simulink model "Gen_nl"  (R2018b)
settings: Solver=FixedStepAuto  StartTime=0.0  StopTime=100  FixedStep=0.1  RelTol=1e-3
undefined symbols (not defined in the file): g, Jx, Jy, Jz, m, phi_DoS_duration, phi_FDI_value, phi_Replay_delay, psi_DoS_duration, psi_FDI_value, psi_Replay_delay, T_DoS_duration, T_FDI_value, T_Replay_delay, tau_phi_DoS_duration, tau_phi_FDI_value, tau_phi_Replay_delay, tau_psi_DoS_duration, tau_psi_FDI_value, tau_psi_Replay_delay, tau_theta_DoS_duration, tau_theta_FDI_value, tau_theta_Replay_delay, theta_DoS_duration, theta_FDI_value, theta_Replay_delay, x_DoS_duration, x_FDI_value, x_Replay_delay, y_DoS_duration, y_FDI_value, y_Replay_delay, z_DoS_duration, z_FDI_value, z_Replay_delay
libraries: simulink x6
settings Model: Creator=afsha  LastModifiedBy=afsha
settings DataIOCC: ReturnWorkspaceOutputs=on  ReturnWorkspaceOutputsName=logsout

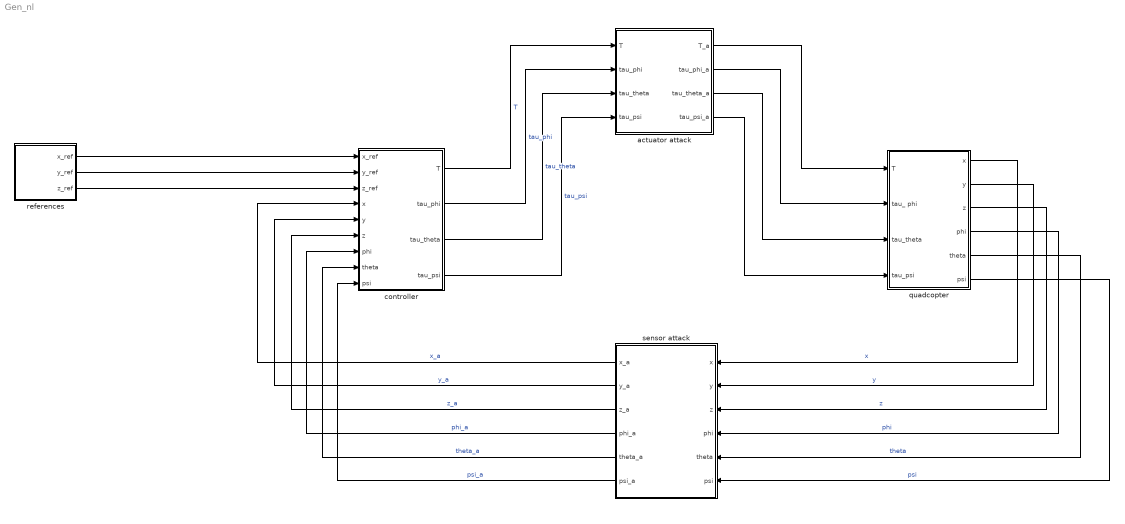
== system Gen_nl ==
  actuator attack : Subsystem
  controller : Subsystem
  quadcopter : Subsystem
  references : Subsystem
  sensor attack : Subsystem
  wires:
  quadcopter/1(x) -> sensor attack/1(x)  "x"
  quadcopter/2(y) -> sensor attack/2(y)  "y"
  quadcopter/3(z) -> sensor attack/3(z)  "z"
  quadcopter/4(phi) -> sensor attack/4(phi)  "phi"
  quadcopter/5(theta) -> sensor attack/5(theta)  "theta"
  quadcopter/6(psi) -> sensor attack/6(psi)  "psi"
  references/1(x_ref) -> controller/1(x_ref)
  references/2(y_ref) -> controller/2(y_ref)
  references/3(z_ref) -> controller/3(z_ref)
  controller/1(T) -> actuator attack/1(T)  "T"
  controller/2(tau_phi) -> actuator attack/2(tau_phi)  "tau_phi"
  controller/3(tau_theta) -> actuator attack/3(tau_theta)  "tau_theta"
  controller/4(tau_psi) -> actuator attack/4(tau_psi)  "tau_psi"
  actuator attack/1(T_a) -> quadcopter/1(T)
  actuator attack/2(tau_phi_a) -> quadcopter/2(tau_ phi)
  actuator attack/3(tau_theta_a) -> quadcopter/3(tau_theta)
  actuator attack/4(tau_psi_a) -> quadcopter/4(tau_psi)
  sensor attack/1(x_a) -> controller/4(x)  "x_a"
  sensor attack/2(y_a) -> controller/5(y)  "y_a"
  sensor attack/3(z_a) -> controller/6(z)  "z_a"
  sensor attack/4(phi_a) -> controller/7(phi)  "phi_a"
  sensor attack/5(theta_a) -> controller/8(theta)  "theta_a"
  sensor attack/6(psi_a) -> controller/9(psi)  "psi_a"

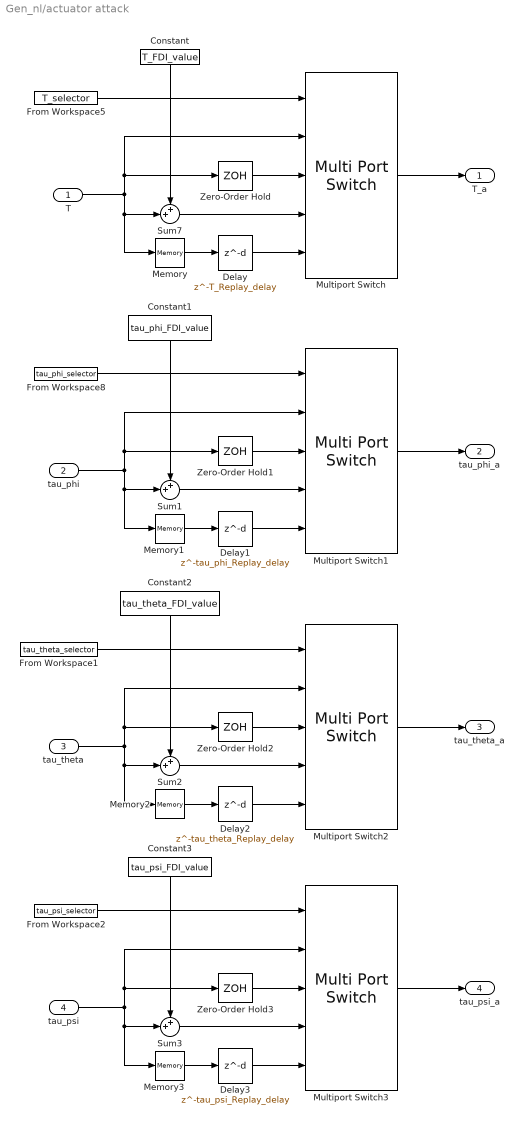
== system Gen_nl/actuator attack ==
  T : Inport
  tau_phi : Inport  Port=2
  tau_theta : Inport  Port=3
  tau_psi : Inport  Port=4
  Constant : Constant  Value=T_FDI_value
  Constant1 : Constant  Value=tau_phi_FDI_value
  Constant2 : Constant  Value=tau_theta_FDI_value
  Constant3 : Constant  Value=tau_psi_FDI_value
  Delay : Delay  DelayLength=T_Replay_delay  DelayLengthUpperLimit=40
  Delay1 : Delay  DelayLength=tau_phi_Replay_delay  DelayLengthUpperLimit=40
  Delay2 : Delay  DelayLength=tau_theta_Replay_delay  DelayLengthUpperLimit=40
  Delay3 : Delay  DelayLength=tau_psi_Replay_delay  DelayLengthUpperLimit=40
  From Workspace1 : FromWorkspace  VariableName=tau_theta_selector  SampleTime=0
  From Workspace2 : FromWorkspace  VariableName=tau_psi_selector  SampleTime=0
  From Workspace5 : FromWorkspace  VariableName=T_selector  SampleTime=0
  From Workspace8 : FromWorkspace  VariableName=tau_phi_selector  SampleTime=0
  Memory{,1..3} (4 alike) : Memory
  Multiport Switch{,1..3} (4 alike) : MultiPortSwitch  Inputs=4
  Sum{1..3,7} (4 alike) : Sum  Inputs=++|
  Zero-Order Hold : ZeroOrderHold  SampleTime=T_DoS_duration
  Zero-Order Hold1 : ZeroOrderHold  SampleTime=tau_phi_DoS_duration
  Zero-Order Hold2 : ZeroOrderHold  SampleTime=tau_theta_DoS_duration
  Zero-Order Hold3 : ZeroOrderHold  SampleTime=tau_psi_DoS_duration
  T_a : Outport
  tau_phi_a : Outport  Port=2
  tau_theta_a : Outport  Port=3
  tau_psi_a : Outport  Port=4
  wires:
  T/1 -> Sum7/2, Memory/1, Multiport Switch/2, Zero-Order Hold/1
  Zero-Order Hold/1 -> Multiport Switch/3
  Sum7/1 -> Multiport Switch/4
  From Workspace5/1 -> Multiport Switch/1
  Multiport Switch/1 -> T_a/1
  Memory/1 -> Delay/1
  Constant/1 -> Sum7/1
  Delay/1 -> Multiport Switch/5
  Memory1/1 -> Delay1/1
  Delay1/1 -> Multiport Switch1/5
  Zero-Order Hold1/1 -> Multiport Switch1/3
  Constant1/1 -> Sum1/1
  Sum1/1 -> Multiport Switch1/4
  Multiport Switch1/1 -> tau_phi_a/1
  tau_phi/1 -> Sum1/2, Memory1/1, Multiport Switch1/2, Zero-Order Hold1/1
  From Workspace8/1 -> Multiport Switch1/1
  Memory2/1 -> Delay2/1
  Delay2/1 -> Multiport Switch2/5
  Zero-Order Hold2/1 -> Multiport Switch2/3
  Constant2/1 -> Sum2/1
  Sum2/1 -> Multiport Switch2/4
  Multiport Switch2/1 -> tau_theta_a/1
  tau_theta/1 -> Sum2/2, Memory2/1, Multiport Switch2/2, Zero-Order Hold2/1
  From Workspace1/1 -> Multiport Switch2/1
  Memory3/1 -> Delay3/1
  Delay3/1 -> Multiport Switch3/5
  Zero-Order Hold3/1 -> Multiport Switch3/3
  Constant3/1 -> Sum3/1
  Sum3/1 -> Multiport Switch3/4
  Multiport Switch3/1 -> tau_psi_a/1
  tau_psi/1 -> Sum3/2, Memory3/1, Multiport Switch3/2, Zero-Order Hold3/1
  From Workspace2/1 -> Multiport Switch3/1

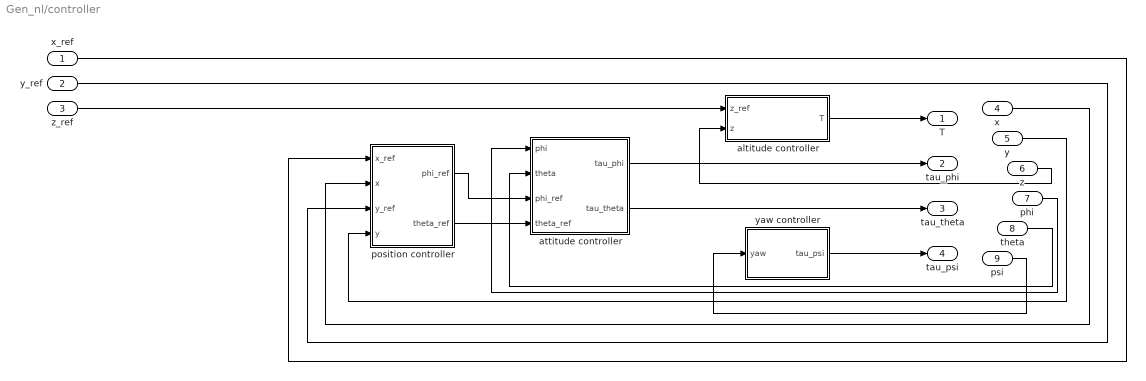
== system Gen_nl/controller ==
  x_ref : Inport
  y_ref : Inport  Port=2
  z_ref : Inport  Port=3
  x : Inport  Port=4
  y : Inport  Port=5
  z : Inport  Port=6
  phi : Inport  Port=7
  theta : Inport  Port=8
  psi : Inport  Port=9
  altitude controller : Subsystem
  attitude controller : Subsystem
  position controller : Subsystem
  yaw controller : Subsystem
  T : Outport
  tau_phi : Outport  Port=2
  tau_theta : Outport  Port=3
  tau_psi : Outport  Port=4
  wires:
  yaw controller/1(tau_psi) -> tau_psi/1
  phi/1 -> attitude controller/1(phi)
  y_ref/1 -> position controller/3(y_ref)
  x/1 -> position controller/2(x)
  position controller/2(theta_ref) -> attitude controller/4(theta_ref)
  position controller/1(phi_ref) -> attitude controller/3(phi_ref)
  x_ref/1 -> position controller/1(x_ref)
  attitude controller/1(tau_phi) -> tau_phi/1
  y/1 -> position controller/4(y)
  psi/1 -> yaw controller/1(yaw)
  attitude controller/2(tau_theta) -> tau_theta/1
  theta/1 -> attitude controller/2(theta)
  z_ref/1 -> altitude controller/1(z_ref)
  altitude controller/1(T) -> T/1
  z/1 -> altitude controller/2(z)

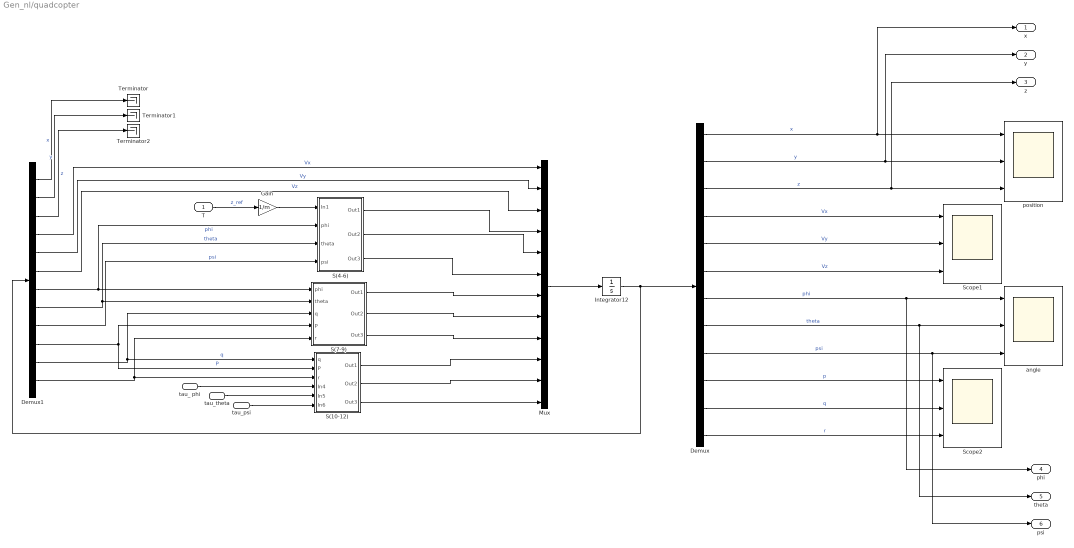
== system Gen_nl/quadcopter ==
  T : Inport
  tau_ phi : Inport  Port=2
  tau_theta : Inport  Port=3
  tau_psi : Inport  Port=4
  Demux : Demux  Outputs=12
  Demux1 : Demux  Outputs=12
  Gain : Gain  Gain=1/m
  Integrator12 : Integrator
  Mux : Mux  Inputs=12
  S(10-12) : Subsystem
  S(4-6) : Subsystem
  S(7-9) : Subsystem
  Scope1 : Scope  NumInputPorts=3
  Scope2 : Scope  NumInputPorts=3
  Terminator : Terminator
  Terminator1 : Terminator
  Terminator2 : Terminator
  angle : Scope  NumInputPorts=3
  position : Scope  NumInputPorts=3
  x : Outport
  y : Outport  Port=2
  z : Outport  Port=3
  phi : Outport  Port=4
  theta : Outport  Port=5
  psi : Outport  Port=6
  wires:
  Mux/1 -> Integrator12/1
  Integrator12/1 -> Demux/1, Demux1/1
  Demux/2 -> position/2, y/1  "y"
  Demux/3 -> z/1, position/3  "z"
  Demux/1 -> x/1, position/1  "x"
  Demux/5 -> Scope1/2  "Vy"
  Demux/4 -> Scope1/1  "Vx"
  Demux/6 -> Scope1/3  "Vz"
  Demux/8 -> angle/2, theta/1  "theta"
  Demux/7 -> angle/1, phi/1  "phi"
  Demux/9 -> angle/3, psi/1  "psi"
  Demux/12 -> Scope2/3  "r"
  Demux/10 -> Scope2/1  "p"
  Demux/11 -> Scope2/2  "q"
  Demux1/4 -> Mux/1  "Vx"
  Demux1/5 -> Mux/2  "Vy"
  Demux1/6 -> Mux/3  "Vz"
  Demux1/8 -> S(4-6)/3(theta), S(7-9)/2(theta)  "theta"
  Demux1/7 -> S(4-6)/2(phi), S(7-9)/1(phi)  "phi"
  Demux1/10 -> S(10-12)/2(P), S(7-9)/4(P)  "P"
  Demux1/11 -> S(7-9)/3(q), S(10-12)/1(q)  "q"
  Demux1/12 -> S(7-9)/5(r), S(10-12)/3(r)
  Gain/1 -> S(4-6)/1(In1)
  Demux1/9 -> S(4-6)/4(psi)  "psi"
  S(4-6)/1(Out1) -> Mux/4
  S(4-6)/2(Out2) -> Mux/5
  S(4-6)/3(Out3) -> Mux/6
  S(7-9)/1(Out1) -> Mux/7
  S(7-9)/2(Out2) -> Mux/8
  S(7-9)/3(Out3) -> Mux/9
  tau_ phi/1 -> S(10-12)/4(In4)
  tau_theta/1 -> S(10-12)/5(In5)
  tau_psi/1 -> S(10-12)/6(In6)
  S(10-12)/1(Out1) -> Mux/10
  S(10-12)/2(Out2) -> Mux/11
  S(10-12)/3(Out3) -> Mux/12
  Demux1/1 -> Terminator/1  "x"
  Demux1/2 -> Terminator1/1  "y"
  Demux1/3 -> Terminator2/1  "z"
  T/1 -> Gain/1  "z_ref"

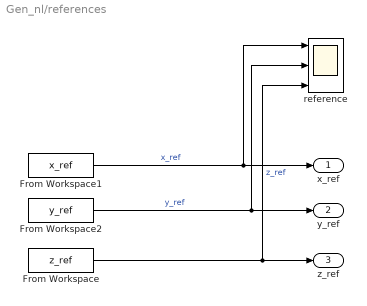
== system Gen_nl/references ==
  From Workspace : FromWorkspace  VariableName=z_ref  SampleTime=0
  From Workspace1 : FromWorkspace  VariableName=x_ref  SampleTime=0
  From Workspace2 : FromWorkspace  VariableName=y_ref  SampleTime=0
  reference : Scope  NumInputPorts=3
  x_ref : Outport
  y_ref : Outport  Port=2
  z_ref : Outport  Port=3
  wires:
  From Workspace1/1 -> reference/1, x_ref/1  "x_ref"
  From Workspace/1 -> reference/3, z_ref/1  "z_ref"
  From Workspace2/1 -> reference/2, y_ref/1  "y_ref"

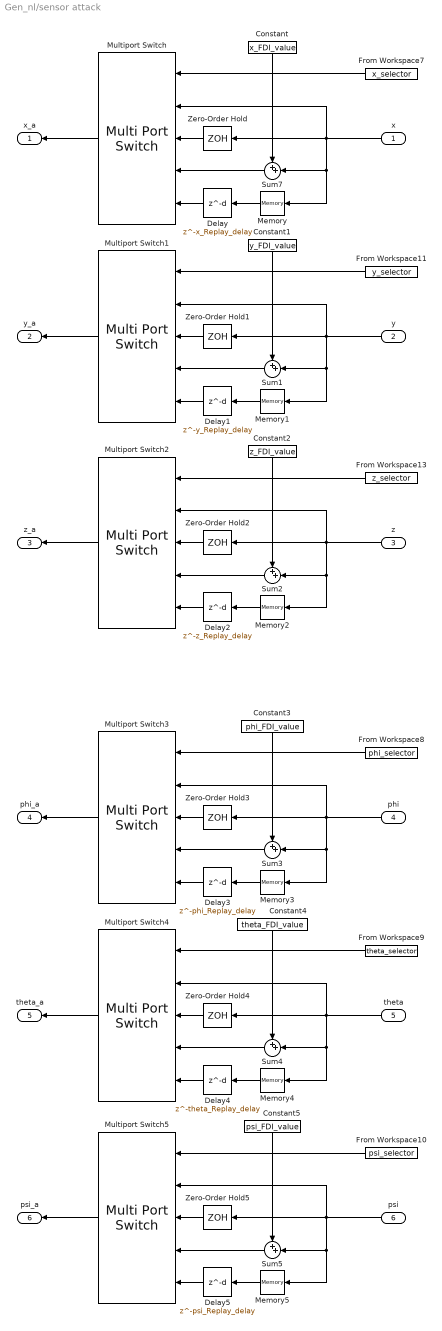
== system Gen_nl/sensor attack ==
  x : Inport
  y : Inport  Port=2
  z : Inport  Port=3
  phi : Inport  Port=4
  theta : Inport  Port=5
  psi : Inport  Port=6
  Constant : Constant  Value=x_FDI_value
  Constant1 : Constant  Value=y_FDI_value
  Constant2 : Constant  Value=z_FDI_value
  Constant3 : Constant  Value=phi_FDI_value
  Constant4 : Constant  Value=theta_FDI_value
  Constant5 : Constant  Value=psi_FDI_value
  Delay : Delay  DelayLength=x_Replay_delay  DelayLengthUpperLimit=40
  Delay1 : Delay  DelayLength=y_Replay_delay  DelayLengthUpperLimit=40
  Delay2 : Delay  DelayLength=z_Replay_delay  DelayLengthUpperLimit=40
  Delay3 : Delay  DelayLength=phi_Replay_delay  DelayLengthUpperLimit=40
  Delay4 : Delay  DelayLength=theta_Replay_delay  DelayLengthUpperLimit=40
  Delay5 : Delay  DelayLength=psi_Replay_delay  DelayLengthUpperLimit=40
  From Workspace10 : FromWorkspace  VariableName=psi_selector  SampleTime=0
  From Workspace11 : FromWorkspace  VariableName=y_selector  SampleTime=0
  From Workspace13 : FromWorkspace  VariableName=z_selector  SampleTime=0
  From Workspace7 : FromWorkspace  VariableName=x_selector  SampleTime=0
  From Workspace8 : FromWorkspace  VariableName=phi_selector  SampleTime=0
  From Workspace9 : FromWorkspace  VariableName=theta_selector  SampleTime=0
  Memory{,1..5} (6 alike) : Memory
  Multiport Switch{,1..5} (6 alike) : MultiPortSwitch  Inputs=4
  Sum{1..5,7} (6 alike) : Sum  Inputs=++|
  Zero-Order Hold : ZeroOrderHold  SampleTime=x_DoS_duration
  Zero-Order Hold1 : ZeroOrderHold  SampleTime=y_DoS_duration
  Zero-Order Hold2 : ZeroOrderHold  SampleTime=z_DoS_duration
  Zero-Order Hold3 : ZeroOrderHold  SampleTime=phi_DoS_duration
  Zero-Order Hold4 : ZeroOrderHold  SampleTime=theta_DoS_duration
  Zero-Order Hold5 : ZeroOrderHold  SampleTime=psi_DoS_duration
  x_a : Outport
  y_a : Outport  Port=2
  z_a : Outport  Port=3
  phi_a : Outport  Port=4
  theta_a : Outport  Port=5
  psi_a : Outport  Port=6
  wires:
  Memory/1 -> Delay/1
  Delay/1 -> Multiport Switch/5
  Zero-Order Hold/1 -> Multiport Switch/3
  Constant/1 -> Sum7/1
  Sum7/1 -> Multiport Switch/4
  Multiport Switch/1 -> x_a/1
  x/1 -> Multiport Switch/2, Zero-Order Hold/1, Sum7/2, Memory/1
  From Workspace7/1 -> Multiport Switch/1
  From Workspace11/1 -> Multiport Switch1/1
  Sum1/1 -> Multiport Switch1/4
  Delay1/1 -> Multiport Switch1/5
  Constant1/1 -> Sum1/1
  Memory1/1 -> Delay1/1
  y/1 -> Multiport Switch1/2, Zero-Order Hold1/1, Sum1/2, Memory1/1
  Multiport Switch1/1 -> y_a/1
  Zero-Order Hold1/1 -> Multiport Switch1/3
  From Workspace13/1 -> Multiport Switch2/1
  Sum2/1 -> Multiport Switch2/4
  Delay2/1 -> Multiport Switch2/5
  Constant2/1 -> Sum2/1
  Memory2/1 -> Delay2/1
  z/1 -> Multiport Switch2/2, Zero-Order Hold2/1, Sum2/2, Memory2/1
  Multiport Switch2/1 -> z_a/1
  Zero-Order Hold2/1 -> Multiport Switch2/3
  From Workspace8/1 -> Multiport Switch3/1
  Sum3/1 -> Multiport Switch3/4
  Delay3/1 -> Multiport Switch3/5
  Constant3/1 -> Sum3/1
  Memory3/1 -> Delay3/1
  phi/1 -> Multiport Switch3/2, Zero-Order Hold3/1, Sum3/2, Memory3/1
  Multiport Switch3/1 -> phi_a/1
  Zero-Order Hold3/1 -> Multiport Switch3/3
  From Workspace9/1 -> Multiport Switch4/1
  Sum4/1 -> Multiport Switch4/4
  Delay4/1 -> Multiport Switch4/5
  Constant4/1 -> Sum4/1
  Memory4/1 -> Delay4/1
  theta/1 -> Multiport Switch4/2, Zero-Order Hold4/1, Sum4/2, Memory4/1
  Multiport Switch4/1 -> theta_a/1
  Zero-Order Hold4/1 -> Multiport Switch4/3
  From Workspace10/1 -> Multiport Switch5/1
  Sum5/1 -> Multiport Switch5/4
  Delay5/1 -> Multiport Switch5/5
  Constant5/1 -> Sum5/1
  Memory5/1 -> Delay5/1
  psi/1 -> Multiport Switch5/2, Zero-Order Hold5/1, Sum5/2, Memory5/1
  Multiport Switch5/1 -> psi_a/1
  Zero-Order Hold5/1 -> Multiport Switch5/3

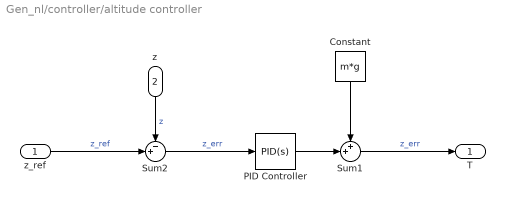
== system Gen_nl/controller/altitude controller ==
  z_ref : Inport
  z : Inport  Port=2
  Constant : Constant  Value=m*g
  PID Controller : simulink/Continuous/PID Controller  Controller=PID  Form=Parallel  TimeDomain=Continuous-time  SampleTime=-1  IntegratorMethod=Forward Euler  FilterMethod=Forward Euler  ControllerParametersSource=internal  P=0.995151437850186  I=0.128436617904908  D=1.76652121748459  UseFilter=on  N=3.43027649580308  TunerSelectOption=Transfer Function Based (PID Tuner App)  InitialConditionSource=internal  InitialConditionForIntegrator=0  InitialConditionForFilter=0  DifferentiatorICPrevScaledInput=0  ExternalReset=none  TrackingMode=off  Kt=1  LimitOutput=off  UpperSaturationLimit=inf  LowerSaturationLimit=-inf  LinearizeAsGain=on  AntiWindupMode=none  Kb=1  POutMin=[]  POutMax=[]  IOutMin=[]  IOutMax=[]  DOutMin=[]  DOutMax=[]  NOutMin=[]  NOutMax=[]  SumOutMin=[]  SumOutMax=[]  SaturationOutMin=[]  SaturationOutMax=[]  PParamMin=[]  PParamMax=[]  IParamMin=[]  IParamMax=[]  DParamMin=[]  DParamMax=[]  NParamMin=[]  NParamMax=[]  KbParamMin=[]  KbParamMax=[]  KtParamMin=[]  KtParamMax=[]  KbOutMin=[]  KbOutMax=[]  KtOutMin=[]  KtOutMax=[]  IntegratorOutMin=[]  IntegratorOutMax=[]  FilterOutMin=[]  FilterOutMax=[]  SumI1OutMin=[]  SumI1OutMax=[]  SumI2OutMin=[]  SumI2OutMax=[]  SumI3OutMin=[]  SumI3OutMax=[]  SumI4OutMin=[]  SumI4OutMax=[]  SumDOutMin=[]  SumDOutMax=[]  DifferentiatorOutMin=[]  DifferentiatorOutMax=[]  FilterDiffOutCoefMin=[]  FilterDiffOutCoefMax=[]  ReciprocalOutMin=[]  ReciprocalOutMax=[]  SumDenOutMin=[]  SumDenOutMax=[]  SumNumOutMin=[]  SumNumOutMax=[]  DivideOutMin=[]  DivideOutMax=[]  IntegratorContinuousStateAttributes=''  IntegratorStateMustResolveToSignalObject=off  IntegratorRTWStateStorageClass=Auto  FilterContinuousStateAttributes=''  FilterStateMustResolveToSignalObject=off  FilterRTWStateStorageClass=Auto  ParallelPVariant=InternalParameters  IdealPVariant=Disabled  IVariant=InternalParameters  DVariant=InternalParameters  IntegratorVariant=Continuous  SatVariant=Disabled  AWVariant=Passthrough  PCopyVariant=Disabled  TRVariant=Disabled  FdbkBlocksVariant=Forward  IdealPFdbkVariant=Disabled  SatFdbkVariant=Disabled  DerivativeFilterVariant=ContFilter  NVariant=InternalParameters  NCopyVariant=Disabled  FilterICVariant=InternalICsFilter  IntegratorICVariant=InternalICs  ExternalResetVariant=Disabled  TRSumVariant=Passthrough  SumFdbkVariant=Disabled  SumVariant=Sum_PID
  Sum1 : Sum  Inputs=++|
  Sum2 : Sum  Inputs=-+|
  T : Outport
  wires:
  z_ref/1 -> Sum2/2  "z_ref"
  Sum2/1 -> PID Controller/1  "z_err"
  z/1 -> Sum2/1  "z"
  PID Controller/1 -> Sum1/2
  Sum1/1 -> T/1  "z_err"
  Constant/1 -> Sum1/1

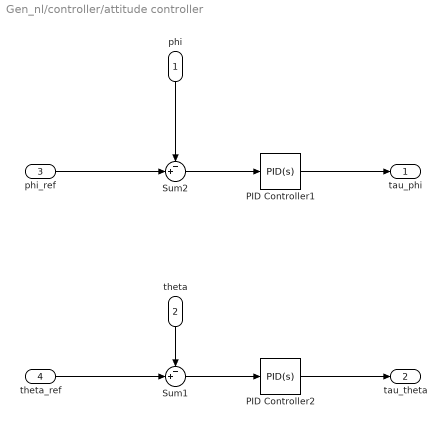
== system Gen_nl/controller/attitude controller ==
  phi : Inport
  theta : Inport  Port=2
  phi_ref : Inport  Port=3
  theta_ref : Inport  Port=4
  PID Controller1 : simulink/Continuous/PID Controller  Controller=PID  Form=Parallel  TimeDomain=Continuous-time  SampleTime=-1  IntegratorMethod=Forward Euler  FilterMethod=Forward Euler  ControllerParametersSource=internal  P=0.00283727985172173  I=0.000300746607233676  D=0.00592713753900793  UseFilter=on  N=3.27588862149554  TunerSelectOption=Transfer Function Based (PID Tuner App)  InitialConditionSource=internal  InitialConditionForIntegrator=0  InitialConditionForFilter=0  DifferentiatorICPrevScaledInput=0  ExternalReset=none  TrackingMode=off  Kt=1  LimitOutput=off  UpperSaturationLimit=inf  LowerSaturationLimit=-inf  LinearizeAsGain=on  AntiWindupMode=none  Kb=1  POutMin=[]  POutMax=[]  IOutMin=[]  IOutMax=[]  DOutMin=[]  DOutMax=[]  NOutMin=[]  NOutMax=[]  SumOutMin=[]  SumOutMax=[]  SaturationOutMin=[]  SaturationOutMax=[]  PParamMin=[]  PParamMax=[]  IParamMin=[]  IParamMax=[]  DParamMin=[]  DParamMax=[]  NParamMin=[]  NParamMax=[]  KbParamMin=[]  KbParamMax=[]  KtParamMin=[]  KtParamMax=[]  KbOutMin=[]  KbOutMax=[]  KtOutMin=[]  KtOutMax=[]  IntegratorOutMin=[]  IntegratorOutMax=[]  FilterOutMin=[]  FilterOutMax=[]  SumI1OutMin=[]  SumI1OutMax=[]  SumI2OutMin=[]  SumI2OutMax=[]  SumI3OutMin=[]  SumI3OutMax=[]  SumI4OutMin=[]  SumI4OutMax=[]  SumDOutMin=[]  SumDOutMax=[]  DifferentiatorOutMin=[]  DifferentiatorOutMax=[]  FilterDiffOutCoefMin=[]  FilterDiffOutCoefMax=[]  ReciprocalOutMin=[]  ReciprocalOutMax=[]  SumDenOutMin=[]  SumDenOutMax=[]  SumNumOutMin=[]  SumNumOutMax=[]  DivideOutMin=[]  DivideOutMax=[]  IntegratorContinuousStateAttributes=''  IntegratorStateMustResolveToSignalObject=off  IntegratorRTWStateStorageClass=Auto  FilterContinuousStateAttributes=''  FilterStateMustResolveToSignalObject=off  FilterRTWStateStorageClass=Auto  ParallelPVariant=InternalParameters  IdealPVariant=Disabled  IVariant=InternalParameters  DVariant=InternalParameters  IntegratorVariant=Continuous  SatVariant=Disabled  AWVariant=Passthrough  PCopyVariant=Disabled  TRVariant=Disabled  FdbkBlocksVariant=Forward  IdealPFdbkVariant=Disabled  SatFdbkVariant=Disabled  DerivativeFilterVariant=ContFilter  NVariant=InternalParameters  NCopyVariant=Disabled  FilterICVariant=InternalICsFilter  IntegratorICVariant=InternalICs  ExternalResetVariant=Disabled  TRSumVariant=Passthrough  SumFdbkVariant=Disabled  SumVariant=Sum_PID
  PID Controller2 : simulink/Continuous/PID Controller  Controller=PID  Form=Parallel  TimeDomain=Continuous-time  SampleTime=-1  IntegratorMethod=Forward Euler  FilterMethod=Forward Euler  ControllerParametersSource=internal  P=0.00376352907272366  I=0.000541941810599823  D=0.00599672187002239  UseFilter=on  N=3.43027649580308  TunerSelectOption=Transfer Function Based (PID Tuner App)  InitialConditionSource=internal  InitialConditionForIntegrator=0  InitialConditionForFilter=0  DifferentiatorICPrevScaledInput=0  ExternalReset=none  TrackingMode=off  Kt=1  LimitOutput=off  UpperSaturationLimit=inf  LowerSaturationLimit=-inf  LinearizeAsGain=on  AntiWindupMode=none  Kb=1  POutMin=[]  POutMax=[]  IOutMin=[]  IOutMax=[]  DOutMin=[]  DOutMax=[]  NOutMin=[]  NOutMax=[]  SumOutMin=[]  SumOutMax=[]  SaturationOutMin=[]  SaturationOutMax=[]  PParamMin=[]  PParamMax=[]  IParamMin=[]  IParamMax=[]  DParamMin=[]  DParamMax=[]  NParamMin=[]  NParamMax=[]  KbParamMin=[]  KbParamMax=[]  KtParamMin=[]  KtParamMax=[]  KbOutMin=[]  KbOutMax=[]  KtOutMin=[]  KtOutMax=[]  IntegratorOutMin=[]  IntegratorOutMax=[]  FilterOutMin=[]  FilterOutMax=[]  SumI1OutMin=[]  SumI1OutMax=[]  SumI2OutMin=[]  SumI2OutMax=[]  SumI3OutMin=[]  SumI3OutMax=[]  SumI4OutMin=[]  SumI4OutMax=[]  SumDOutMin=[]  SumDOutMax=[]  DifferentiatorOutMin=[]  DifferentiatorOutMax=[]  FilterDiffOutCoefMin=[]  FilterDiffOutCoefMax=[]  ReciprocalOutMin=[]  ReciprocalOutMax=[]  SumDenOutMin=[]  SumDenOutMax=[]  SumNumOutMin=[]  SumNumOutMax=[]  DivideOutMin=[]  DivideOutMax=[]  IntegratorContinuousStateAttributes=''  IntegratorStateMustResolveToSignalObject=off  IntegratorRTWStateStorageClass=Auto  FilterContinuousStateAttributes=''  FilterStateMustResolveToSignalObject=off  FilterRTWStateStorageClass=Auto  ParallelPVariant=InternalParameters  IdealPVariant=Disabled  IVariant=InternalParameters  DVariant=InternalParameters  IntegratorVariant=Continuous  SatVariant=Disabled  AWVariant=Passthrough  PCopyVariant=Disabled  TRVariant=Disabled  FdbkBlocksVariant=Forward  IdealPFdbkVariant=Disabled  SatFdbkVariant=Disabled  DerivativeFilterVariant=ContFilter  NVariant=InternalParameters  NCopyVariant=Disabled  FilterICVariant=InternalICsFilter  IntegratorICVariant=InternalICs  ExternalResetVariant=Disabled  TRSumVariant=Passthrough  SumFdbkVariant=Disabled  SumVariant=Sum_PID
  Sum1 : Sum  Inputs=-+|
  Sum2 : Sum  Inputs=-+|
  tau_phi : Outport
  tau_theta : Outport  Port=2
  wires:
  phi/1 -> Sum2/1
  theta/1 -> Sum1/1
  phi_ref/1 -> Sum2/2
  theta_ref/1 -> Sum1/2
  Sum1/1 -> PID Controller2/1
  PID Controller2/1 -> tau_theta/1
  Sum2/1 -> PID Controller1/1
  PID Controller1/1 -> tau_phi/1

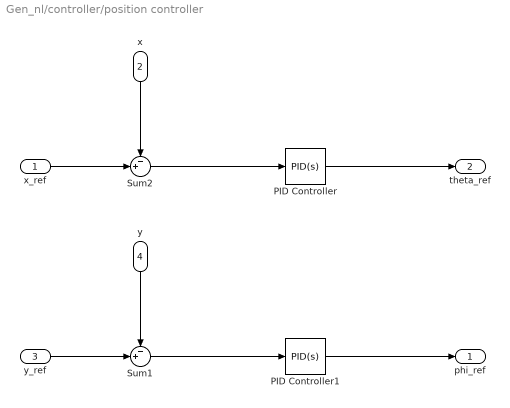
== system Gen_nl/controller/position controller ==
  x_ref : Inport
  x : Inport  Port=2
  y_ref : Inport  Port=3
  y : Inport  Port=4
  PID Controller : simulink/Continuous/PID Controller  Controller=PID  Form=Parallel  TimeDomain=Continuous-time  SampleTime=-1  IntegratorMethod=Forward Euler  FilterMethod=Forward Euler  ControllerParametersSource=internal  P=-0.0353666022144165  I=-0.000286794158433156  D=-0.0628063352706131  UseFilter=on  N=2.54551622754876  TunerSelectOption=Transfer Function Based (PID Tuner App)  InitialConditionSource=internal  InitialConditionForIntegrator=0  InitialConditionForFilter=0  DifferentiatorICPrevScaledInput=0  ExternalReset=none  TrackingMode=off  Kt=1  LimitOutput=off  UpperSaturationLimit=inf  LowerSaturationLimit=-inf  LinearizeAsGain=on  AntiWindupMode=none  Kb=1  POutMin=[]  POutMax=[]  IOutMin=[]  IOutMax=[]  DOutMin=[]  DOutMax=[]  NOutMin=[]  NOutMax=[]  SumOutMin=[]  SumOutMax=[]  SaturationOutMin=[]  SaturationOutMax=[]  PParamMin=[]  PParamMax=[]  IParamMin=[]  IParamMax=[]  DParamMin=[]  DParamMax=[]  NParamMin=[]  NParamMax=[]  KbParamMin=[]  KbParamMax=[]  KtParamMin=[]  KtParamMax=[]  KbOutMin=[]  KbOutMax=[]  KtOutMin=[]  KtOutMax=[]  IntegratorOutMin=[]  IntegratorOutMax=[]  FilterOutMin=[]  FilterOutMax=[]  SumI1OutMin=[]  SumI1OutMax=[]  SumI2OutMin=[]  SumI2OutMax=[]  SumI3OutMin=[]  SumI3OutMax=[]  SumI4OutMin=[]  SumI4OutMax=[]  SumDOutMin=[]  SumDOutMax=[]  DifferentiatorOutMin=[]  DifferentiatorOutMax=[]  FilterDiffOutCoefMin=[]  FilterDiffOutCoefMax=[]  ReciprocalOutMin=[]  ReciprocalOutMax=[]  SumDenOutMin=[]  SumDenOutMax=[]  SumNumOutMin=[]  SumNumOutMax=[]  DivideOutMin=[]  DivideOutMax=[]  IntegratorContinuousStateAttributes=''  IntegratorStateMustResolveToSignalObject=off  IntegratorRTWStateStorageClass=Auto  FilterContinuousStateAttributes=''  FilterStateMustResolveToSignalObject=off  FilterRTWStateStorageClass=Auto  ParallelPVariant=InternalParameters  IdealPVariant=Disabled  IVariant=InternalParameters  DVariant=InternalParameters  IntegratorVariant=Continuous  SatVariant=Disabled  AWVariant=Passthrough  PCopyVariant=Disabled  TRVariant=Disabled  FdbkBlocksVariant=Forward  IdealPFdbkVariant=Disabled  SatFdbkVariant=Disabled  DerivativeFilterVariant=ContFilter  NVariant=InternalParameters  NCopyVariant=Disabled  FilterICVariant=InternalICsFilter  IntegratorICVariant=InternalICs  ExternalResetVariant=Disabled  TRSumVariant=Passthrough  SumFdbkVariant=Disabled  SumVariant=Sum_PID
  PID Controller1 : simulink/Continuous/PID Controller  Controller=PID  Form=Parallel  TimeDomain=Continuous-time  SampleTime=-1  IntegratorMethod=Forward Euler  FilterMethod=Forward Euler  ControllerParametersSource=internal  P=0.0344011339376346  I=0.00030706355489176  D=0.0770084502146799  UseFilter=on  N=2.81850869669594  TunerSelectOption=Transfer Function Based (PID Tuner App)  InitialConditionSource=internal  InitialConditionForIntegrator=0  InitialConditionForFilter=0  DifferentiatorICPrevScaledInput=0  ExternalReset=none  TrackingMode=off  Kt=1  LimitOutput=off  UpperSaturationLimit=inf  LowerSaturationLimit=-inf  LinearizeAsGain=on  AntiWindupMode=none  Kb=1  POutMin=[]  POutMax=[]  IOutMin=[]  IOutMax=[]  DOutMin=[]  DOutMax=[]  NOutMin=[]  NOutMax=[]  SumOutMin=[]  SumOutMax=[]  SaturationOutMin=[]  SaturationOutMax=[]  PParamMin=[]  PParamMax=[]  IParamMin=[]  IParamMax=[]  DParamMin=[]  DParamMax=[]  NParamMin=[]  NParamMax=[]  KbParamMin=[]  KbParamMax=[]  KtParamMin=[]  KtParamMax=[]  KbOutMin=[]  KbOutMax=[]  KtOutMin=[]  KtOutMax=[]  IntegratorOutMin=[]  IntegratorOutMax=[]  FilterOutMin=[]  FilterOutMax=[]  SumI1OutMin=[]  SumI1OutMax=[]  SumI2OutMin=[]  SumI2OutMax=[]  SumI3OutMin=[]  SumI3OutMax=[]  SumI4OutMin=[]  SumI4OutMax=[]  SumDOutMin=[]  SumDOutMax=[]  DifferentiatorOutMin=[]  DifferentiatorOutMax=[]  FilterDiffOutCoefMin=[]  FilterDiffOutCoefMax=[]  ReciprocalOutMin=[]  ReciprocalOutMax=[]  SumDenOutMin=[]  SumDenOutMax=[]  SumNumOutMin=[]  SumNumOutMax=[]  DivideOutMin=[]  DivideOutMax=[]  IntegratorContinuousStateAttributes=''  IntegratorStateMustResolveToSignalObject=off  IntegratorRTWStateStorageClass=Auto  FilterContinuousStateAttributes=''  FilterStateMustResolveToSignalObject=off  FilterRTWStateStorageClass=Auto  ParallelPVariant=InternalParameters  IdealPVariant=Disabled  IVariant=InternalParameters  DVariant=InternalParameters  IntegratorVariant=Continuous  SatVariant=Disabled  AWVariant=Passthrough  PCopyVariant=Disabled  TRVariant=Disabled  FdbkBlocksVariant=Forward  IdealPFdbkVariant=Disabled  SatFdbkVariant=Disabled  DerivativeFilterVariant=ContFilter  NVariant=InternalParameters  NCopyVariant=Disabled  FilterICVariant=InternalICsFilter  IntegratorICVariant=InternalICs  ExternalResetVariant=Disabled  TRSumVariant=Passthrough  SumFdbkVariant=Disabled  SumVariant=Sum_PID
  Sum1 : Sum  Inputs=-+|
  Sum2 : Sum  Inputs=-+|
  phi_ref : Outport
  theta_ref : Outport  Port=2
  wires:
  x_ref/1 -> Sum2/2
  x/1 -> Sum2/1
  Sum2/1 -> PID Controller/1
  PID Controller/1 -> theta_ref/1
  Sum1/1 -> PID Controller1/1
  y_ref/1 -> Sum1/2
  y/1 -> Sum1/1
  PID Controller1/1 -> phi_ref/1

== system Gen_nl/controller/yaw controller ==
  yaw : Inport
  Constant : Constant  Value=0
  PID Controller3 : simulink/Continuous/PID Controller  Controller=PID  Form=Parallel  TimeDomain=Continuous-time  SampleTime=-1  IntegratorMethod=Forward Euler  FilterMethod=Forward Euler  ControllerParametersSource=internal  P=0.00651371850229212  I=0.000840676044468491  D=0.0115626843326264  UseFilter=on  N=3.43027649580308  TunerSelectOption=Transfer Function Based (PID Tuner App)  InitialConditionSource=internal  InitialConditionForIntegrator=0  InitialConditionForFilter=0  DifferentiatorICPrevScaledInput=0  ExternalReset=none  TrackingMode=off  Kt=1  LimitOutput=off  UpperSaturationLimit=inf  LowerSaturationLimit=-inf  LinearizeAsGain=on  AntiWindupMode=none  Kb=1  POutMin=[]  POutMax=[]  IOutMin=[]  IOutMax=[]  DOutMin=[]  DOutMax=[]  NOutMin=[]  NOutMax=[]  SumOutMin=[]  SumOutMax=[]  SaturationOutMin=[]  SaturationOutMax=[]  PParamMin=[]  PParamMax=[]  IParamMin=[]  IParamMax=[]  DParamMin=[]  DParamMax=[]  NParamMin=[]  NParamMax=[]  KbParamMin=[]  KbParamMax=[]  KtParamMin=[]  KtParamMax=[]  KbOutMin=[]  KbOutMax=[]  KtOutMin=[]  KtOutMax=[]  IntegratorOutMin=[]  IntegratorOutMax=[]  FilterOutMin=[]  FilterOutMax=[]  SumI1OutMin=[]  SumI1OutMax=[]  SumI2OutMin=[]  SumI2OutMax=[]  SumI3OutMin=[]  SumI3OutMax=[]  SumI4OutMin=[]  SumI4OutMax=[]  SumDOutMin=[]  SumDOutMax=[]  DifferentiatorOutMin=[]  DifferentiatorOutMax=[]  FilterDiffOutCoefMin=[]  FilterDiffOutCoefMax=[]  ReciprocalOutMin=[]  ReciprocalOutMax=[]  SumDenOutMin=[]  SumDenOutMax=[]  SumNumOutMin=[]  SumNumOutMax=[]  DivideOutMin=[]  DivideOutMax=[]  IntegratorContinuousStateAttributes=''  IntegratorStateMustResolveToSignalObject=off  IntegratorRTWStateStorageClass=Auto  FilterContinuousStateAttributes=''  FilterStateMustResolveToSignalObject=off  FilterRTWStateStorageClass=Auto  ParallelPVariant=InternalParameters  IdealPVariant=Disabled  IVariant=InternalParameters  DVariant=InternalParameters  IntegratorVariant=Continuous  SatVariant=Disabled  AWVariant=Passthrough  PCopyVariant=Disabled  TRVariant=Disabled  FdbkBlocksVariant=Forward  IdealPFdbkVariant=Disabled  SatFdbkVariant=Disabled  DerivativeFilterVariant=ContFilter  NVariant=InternalParameters  NCopyVariant=Disabled  FilterICVariant=InternalICsFilter  IntegratorICVariant=InternalICs  ExternalResetVariant=Disabled  TRSumVariant=Passthrough  SumFdbkVariant=Disabled  SumVariant=Sum_PID
  Sum2 : Sum  Inputs=-+|
  tau_psi : Outport
  wires:
  yaw/1 -> Sum2/1
  Constant/1 -> Sum2/2
  Sum2/1 -> PID Controller3/1
  PID Controller3/1 -> tau_psi/1

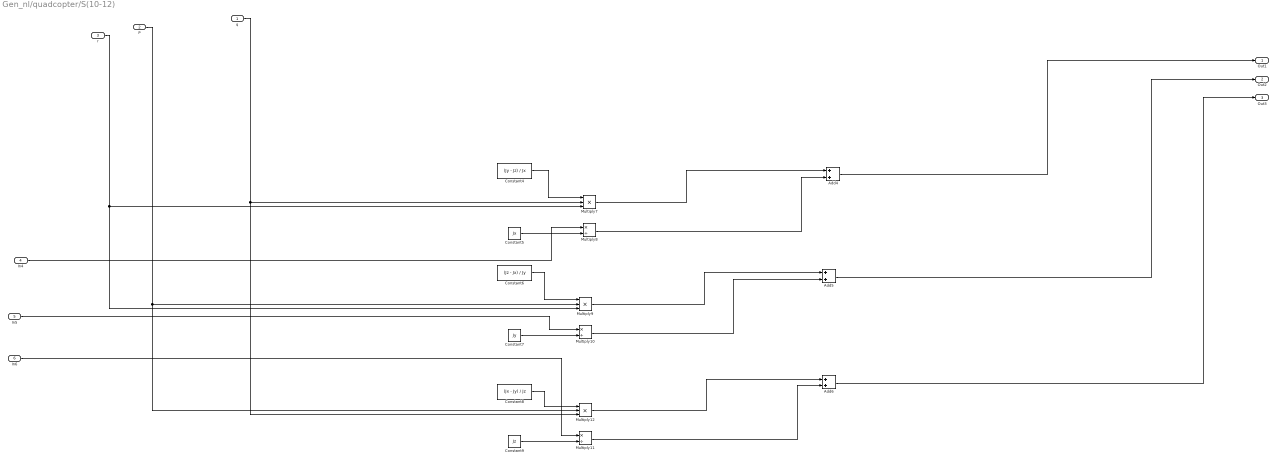
== system Gen_nl/quadcopter/S(10-12) ==
  q : Inport
  P : Inport  Port=2
  r : Inport  Port=3
  In4 : Inport  Port=4
  In5 : Inport  Port=5
  In6 : Inport  Port=6
  Add4 : Sum
  Add5 : Sum
  Add6 : Sum
  Constant4 : Constant  Value=(Jy - Jz) / Jx
  Constant5 : Constant  Value=Jx
  Constant6 : Constant  Value=(Jz - Jx) / Jy
  Constant7 : Constant  Value=Jy
  Constant8 : Constant  Value=(Jx - Jy) / Jz
  Constant9 : Constant  Value=Jz
  Multiply10 : Product  Inputs=*/
  Multiply11 : Product  Inputs=*/
  Multiply12 : Product  Inputs=3
  Multiply7 : Product  Inputs=3
  Multiply8 : Product  Inputs=*/
  Multiply9 : Product  Inputs=3
  Out1 : Outport
  Out2 : Outport  Port=2
  Out3 : Outport  Port=3
  wires:
  r/1 -> Multiply9/3, Multiply7/3
  Constant8/1 -> Multiply12/1
  In5/1 -> Multiply10/1
  Multiply8/1 -> Add4/2
  Multiply7/1 -> Add4/1
  Constant7/1 -> Multiply10/2
  Constant5/1 -> Multiply8/2
  Constant4/1 -> Multiply7/1
  q/1 -> Multiply7/2, Multiply12/3
  Multiply10/1 -> Add5/2
  Multiply9/1 -> Add5/1
  Constant9/1 -> Multiply11/2
  In6/1 -> Multiply11/1
  Constant6/1 -> Multiply9/1
  Multiply12/1 -> Add6/1
  P/1 -> Multiply9/2, Multiply12/2
  In4/1 -> Multiply8/1
  Multiply11/1 -> Add6/2
  Add4/1 -> Out1/1
  Add5/1 -> Out2/1
  Add6/1 -> Out3/1

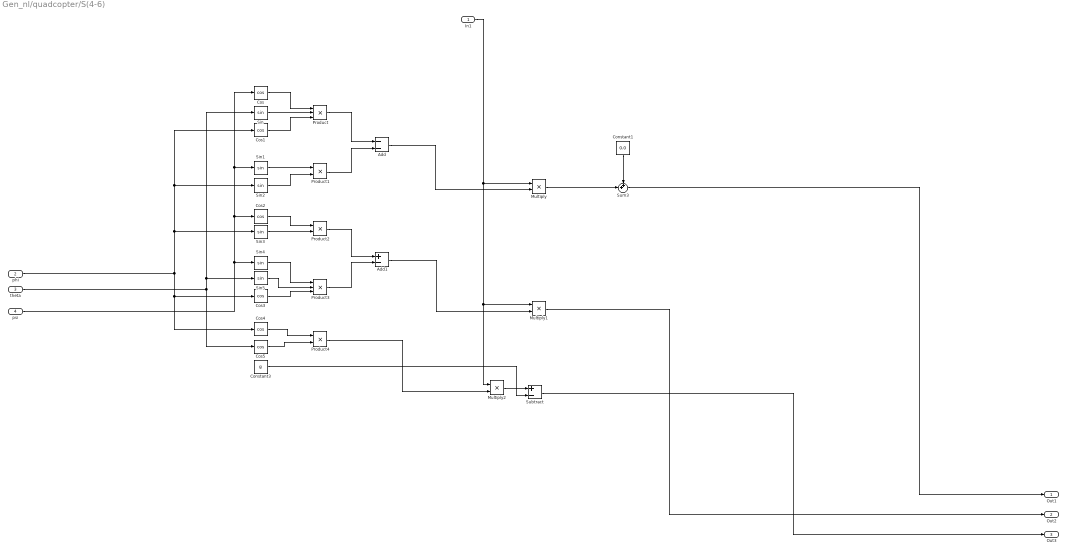
== system Gen_nl/quadcopter/S(4-6) ==
  In1 : Inport
  phi : Inport  Port=2
  theta : Inport  Port=3
  psi : Inport  Port=4
  Add : Sum  Inputs=--
  Add1 : Sum  Inputs=+-
  Constant1 : Constant  Value=0.0
  Constant3 : Constant  Value=g
  Cos{,1..5} (6 alike) : Trigonometry  Operator=cos
  Multiply : Product
  Multiply1 : Product
  Multiply2 : Product
  Product : Product  Inputs=3
  Product1 : Product
  Product2 : Product
  Product3 : Product  Inputs=3
  Product4 : Product
  Sin{,1..5} (6 alike) : Trigonometry
  Subtract : Sum  Inputs=+-
  Sum3 : Sum  Inputs=++|
  Out1 : Outport
  Out2 : Outport  Port=2
  Out3 : Outport  Port=3
  wires:
  phi/1 -> Cos4/1, Cos3/1, Cos1/1, Sin2/1, Sin3/1
  theta/1 -> Sin/1, Sin5/1, Cos5/1
  Sum3/1 -> Out1/1
  Constant1/1 -> Sum3/1
  Product1/1 -> Add/2
  Sin3/1 -> Product2/2
  Cos/1 -> Product/1
  Cos1/1 -> Product/3
  Multiply/1 -> Sum3/2
  Sin/1 -> Product/2
  Cos5/1 -> Product4/2
  psi/1 -> Cos/1, Sin1/1, Cos2/1, Sin4/1
  Cos3/1 -> Product3/3
  Product2/1 -> Add1/1
  Add1/1 -> Multiply1/2
  Sin1/1 -> Product1/1
  Sin4/1 -> Product3/1
  Sin5/1 -> Product3/2
  Cos4/1 -> Product4/1
  Cos2/1 -> Product2/1
  Subtract/1 -> Out3/1
  Sin2/1 -> Product1/2
  Constant3/1 -> Subtract/2
  Product4/1 -> Multiply2/2
  In1/1 -> Multiply2/1, Multiply1/1, Multiply/1
  Add/1 -> Multiply/2
  Product3/1 -> Add1/2
  Multiply2/1 -> Subtract/1
  Product/1 -> Add/1
  Multiply1/1 -> Out2/1

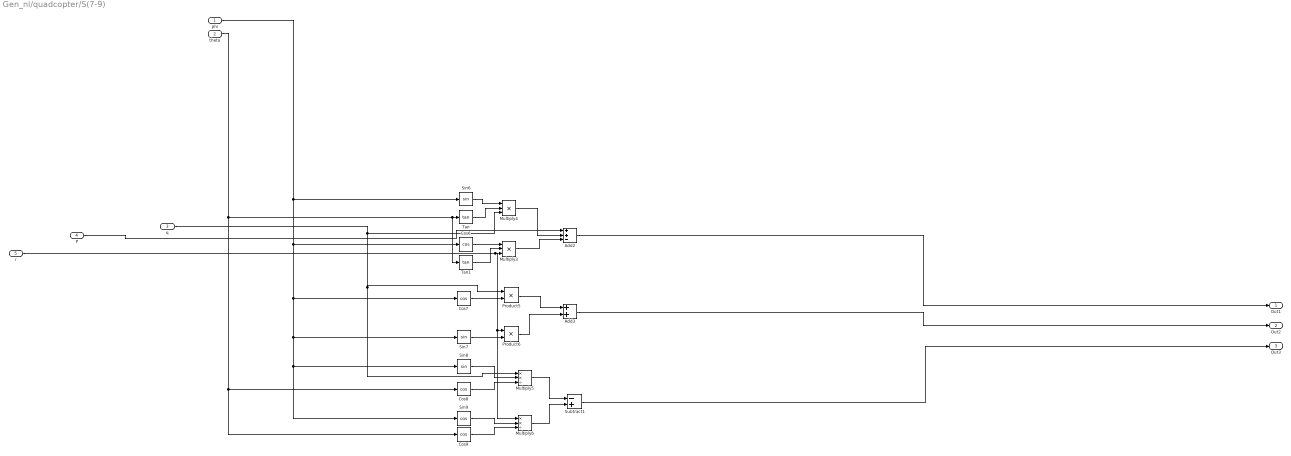
== system Gen_nl/quadcopter/S(7-9) ==
  phi : Inport
  theta : Inport  Port=2
  q : Inport  Port=3
  P : Inport  Port=4
  r : Inport  Port=5
  Add2 : Sum  Inputs=++-
  Add3 : Sum
  Cos{6..9} (4 alike) : Trigonometry  Operator=cos
  Multiply3 : Product  Inputs=3
  Multiply4 : Product  Inputs=3
  Multiply5 : Product  Inputs=**/
  Multiply6 : Product  Inputs=**/
  Product5 : Product
  Product6 : Product
  Sin6 : Trigonometry
  Sin7 : Trigonometry
  Sin8 : Trigonometry
  Sin9 : Trigonometry  Operator=cos
  Subtract1 : Sum  Inputs=-+
  Tan : Trigonometry  Operator=tan
  Tan1 : Trigonometry  Operator=tan
  Out1 : Outport
  Out2 : Outport  Port=2
  Out3 : Outport  Port=3
  wires:
  Multiply5/1 -> Subtract1/1
  q/1 -> Multiply5/1, Product5/1, Multiply4/3
  phi/1 -> Sin9/1, Sin8/1, Sin7/1, Cos7/1, Cos6/1, Sin6/1
  Multiply4/1 -> Add2/2
  theta/1 -> Cos9/1, Cos8/1, Tan/1, Tan1/1
  Tan/1 -> Multiply4/2
  r/1 -> Multiply6/1, Product6/1, Multiply3/3
  Multiply6/1 -> Subtract1/2
  Sin9/1 -> Multiply6/2
  Sin6/1 -> Multiply4/1
  Sin8/1 -> Multiply5/2
  Tan1/1 -> Multiply3/2
  Product5/1 -> Add3/1
  Cos6/1 -> Multiply3/1
  Product6/1 -> Add3/2
  Sin7/1 -> Product6/2
  Multiply3/1 -> Add2/3
  Cos7/1 -> Product5/2
  Cos8/1 -> Multiply5/3
  Cos9/1 -> Multiply6/3
  Subtract1/1 -> Out3/1
  P/1 -> Add2/1
  Add2/1 -> Out1/1
  Add3/1 -> Out2/1
